simulink model "ret2"  (R2013a)
settings: Solver=ode23tb  StartTime=0.0  StopTime=5  RelTol=1e-3
values from neighbouring files (symbols this model uses):
  alfa = 90    [dcmsi.m]
  C = 1    [dcmsi.m]
  J = 1.1e-4    (= 0.00011)    [dcmsi.m]
  kt = 0.038    [dcmsi.m]
  La = 6.67e-4    (= 0.000667)    [dcmsi.m]
  Ra = 1.6    [dcmsi.m]
  V_source = 24*sqrt(2)    [dcmsi.m]
libraries: powerlib x10
settings Model: Creator=dello  LastModifiedBy=dello
settings DataIOCC: SignalLoggingSaveFormat=ModelDataLogs  SignalLoggingName=results
settings OptimizationCC: BlockReduction=off

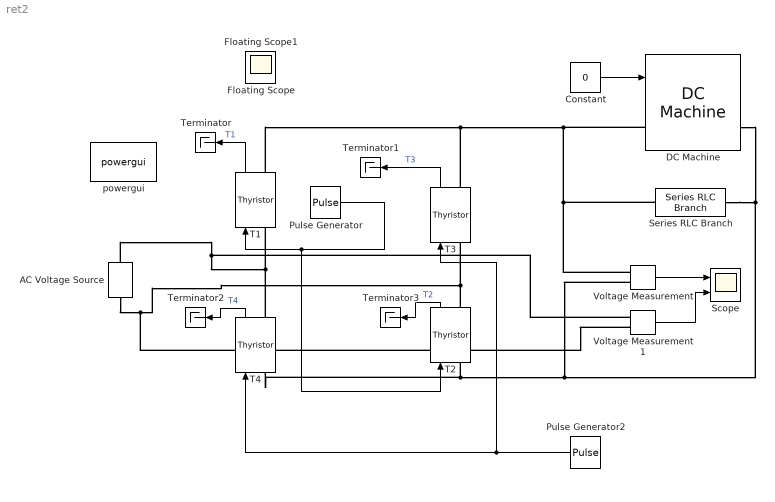
== system ret2 ==
  AC Voltage Source : powerlib/Electrical Sources/AC Voltage Source  Amplitude=V_source  Phase=0  Frequency=60  SampleTime=0  Measurements=Voltage
  Constant : Constant  Value=0
  DC Machine : powerlib/Machines/DC Machine  PresetModel=No  MechanicalLoad=Torque TL  FieldType=Permanent magnet  ShowDetailedParameters=on  RLa="[Ra  La]"  RLf="[ 240  120]"  Laf=1.8  MachineConstant=Torque constant (N.m/A)  Ke=1.8  Kt=kt  J=J  Bm=B  Tf=0  w0=0  Ifinit=1  TsPowergui=0  TsBlock=-1
  Pulse Generator : DiscretePulseGenerator  PulseType=Time based  Period=1/60  PulseWidth=30  PhaseDelay=alfa/360/60
  Pulse Generator2 : DiscretePulseGenerator  PulseType=Time based  Period=1/60  PulseWidth=30  PhaseDelay=(alfa + 180)/360/60
  Scope : Scope  NumInputPorts=2
      settings: TimeRange=5  YMin=-5~-5  YMax=5~5
  Series RLC Branch : powerlib/Elements/Series RLC Branch  LConnTagsString=__new0  RConnTagsString=__new0  BranchType=C  Resistance=1  Inductance=1e-3  SetiL0=off  InitialCurrent=0  Capacitance=C  Setx0=off  InitialVoltage=0  Measurements=None
  T{1..4} (4 alike) : powerlib/Power Electronics/Thyristor  Ron=0.001  Lon=0  Vf=0.8  IC=0  Rs=500  Cs=250e-9  Measurements=on
  Terminator{,1..3} (4 alike) : Terminator
  Voltage Measurement : powerlib/Measurements/Voltage Measurement  PhasorSimulation=off  OutputType=Complex  PSBequivalent=0
  Voltage Measurement1 : powerlib/Measurements/Voltage Measurement  PhasorSimulation=off  OutputType=Complex  PSBequivalent=0
  powergui : powerlib/powergui  Priority=1  SimulationMode=Continuous  SolverType=Tustin  SampleTime=50e-6  frequency=60  SPID=off  DisableSnubberDevices=off  DisableRonSwitches=off  DisableVfSwitches=off  SwTol=0  Interpol=off  DisplayEquations=off  frequencyindice=0  Pbase=100e6  ErrMax=1e-4  Iterations=50  UnitsV=V  UnitsW=W  FunctionMessages=off  echomessages=off  HookPort=off  EnableUseOfTLC=off  x0status=blocks  RestoreLinks=warning  ResistiveCurrentMeasurement=off  Frange=[0:2:500]  Ylog=off  Xlog=on  ShowGrid=off  save=off  variable=ZData  ZoomFFT=off  StartTime=0.0  cycles=1  DisplayStyle=1  fundamental=60  FreqAxis=off  MaxFrequency=1000  frequencyindicesteady=1  RmsSteady=1  display=off  Ts=0  methode=off
  Floating Scope : Scope  NumInputPorts=8
      settings: Floating=on  TimeRange=0.03333333333333333  YMin=-5~-5~-5~-5~-5~-5~-5~-5  YMax=5~5~5~5~5~5~5~5  SaveName=diodes
  Floating Scope1 : Scope
      settings: Floating=on  TimeRange=0.03333333333333333  SaveName=simdata
  wires:
  T1/1 -> Terminator/1  "T1"
  T3/1 -> Terminator1/1  "T3"
  T2/1 -> Terminator3/1  "T2"
  T4/1 -> Terminator2/1  "T4"
  Pulse Generator/1 -> T2/1, T1/1
  Pulse Generator2/1 -> T3/1, T4/1
  Constant/1 -> DC Machine/1
  Voltage Measurement/1 -> Scope/1
  Voltage Measurement1/1 -> Scope/2
  connections:
  AC Voltage Source/RConn1 -- Voltage Measurement1/LConn1 -- T4/RConn1 -- T1/LConn1
  AC Voltage Source/LConn1 -- Voltage Measurement1/LConn2 -- T3/LConn1 -- T2/RConn1
  T3/RConn1 -- Voltage Measurement/LConn1 -- Series RLC Branch/LConn1 -- DC Machine/LConn1 -- T1/RConn1
  T4/LConn1 -- Voltage Measurement/LConn2 -- DC Machine/RConn1 -- Series RLC Branch/RConn1 -- T2/LConn1
